simulink model "VU_testSoundTone3"  (Simulink 10.0)
settings: Solver=FixedStepDiscrete  StartTime=0.0  StopTime=inf  FixedStep=0.1  RelTol=1e-3
libraries: lego_nxt_lib x3
settings Model: Creator=jpeytonj  LastModifiedBy=bhisma
settings DataIOCC: LimitDataPoints=on  SignalLoggingSaveFormat=ModelDataLogs
settings OptimizationCC: ExpressionDepthLimit=2147483647
settings DebuggingCC: SolverPrmCheckMsg=warning  FcnCallInpInsideContextMsg=warning  StateNameClashWarn=warning
settings SFSimCC: SimParseCustomCode=off
settings RTWCC: Description=Lego NXT Real-Time Target  SystemTargetFile=lrt.tlc  GenCodeOnly=on  TemplateMakefile=lrt_ecrobot.tmf
settings STFCustomTargetCC: ModelReferenceCompliant=off  GeneratePreprocessorConditionals=Disable all  MatFileLogging=on  CPPClassGenCompliant=on  SystemTargetFile=lrt.tlc
settings GRTTargetCC: ModelReferenceCompliant=off  ParMdlRefBuildCompliant=off  CompOptLevelCompliant=off  ConcurrentExecutionCompliant=off  GeneratePreprocessorConditionals=Disable all  UseToolchainInfoCompliant=off  ExtModeMexFile=noextcomm
settings CustomProperty: DataType=RTWOptions_EnumType_C__LegoMindstorms_VU-LRT_lrt_1codeGenType  Value=Integer-only
settings EnumStrPairs: String=Integer-only
settings ConfigComp: CovExternalEMLEnable=off

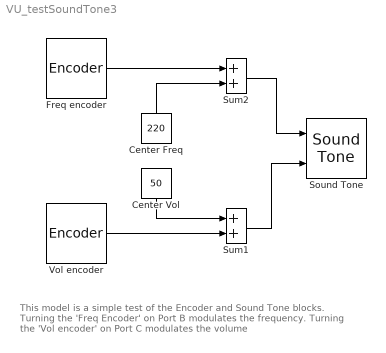
== system VU_testSoundTone3 ==
  note: This model is a simple test of the Encoder and Sound Tone blocks.
      | Turning the 'Freq Encoder' on Port B modulates the frequency.
      | Turning the 'Vol encoder' on Port C modulates the volume
  Center Freq : Constant  Value=220
  Center Vol : Constant  Value=50
  Freq encoder : lego_nxt_lib/Encoder  port=Port B  st=0.1
  Sound Tone : lego_nxt_lib/Sound Tone  SystemSampleTime=-1  freqsrc=External  freq=220  volsrc=External  vol=70
  Sum1 : Sum  OutDataTypeStr=uint8
  Sum2 : Sum  OutDataTypeStr=uint32
  Vol encoder : lego_nxt_lib/Encoder  port=Port C  st=0.1
  wires:
  Sum2/1 -> Sound Tone/1
  Freq encoder/1 -> Sum2/1
  Center Freq/1 -> Sum2/2
  Vol encoder/1 -> Sum1/2
  Center Vol/1 -> Sum1/1
  Sum1/1 -> Sound Tone/2
